simulink model "kcco"  (Simulink 10.0)
settings: Solver=ode45  StartTime=0.0  StopTime=0.05  RelTol=1e-6  EnableMultiTasking=on
settings Model: Creator=mvcmv  LastModifiedBy=mvcmv
settings DataIOCC: LimitDataPoints=on  MaxDataPoints=10000  SignalLoggingSaveFormat=ModelDataLogs  SignalLoggingName=sigsOut
settings OptimizationCC: LifeSpan=auto
settings DebuggingCC: SaveWithParameterizedLinksMsg=none  SignalResolutionControl=TryResolveAllWithWarning  MultiTaskDSMMsg=warning  MultiTaskCondExecSysMsg=none  SFUnexpectedBacktrackingDiag=error  SFNoUnconditionalDefaultTransitionDiag=error  SFExecutionAtInitializationDiag=warning  ArithmeticOperatorsInVariantConditions=error
settings HardwareCC: TargetUnknown=on
settings SFSimCC: SimUseLocalCustomCode=on  CustomCodeUndefinedFunction=FilterOut
settings RTWCC: RTWUseLocalCustomCode=on
settings CodeAppCC: StateflowObjectComments=off
settings GRTTargetCC: TargetLangStandard=C99 (ISO)

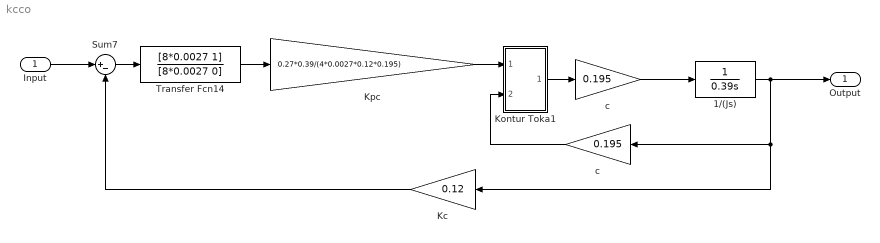
== system kcco ==
  Input : Inport
  1/(Js) : TransferFcn  Denominator=[0.39 0]
  Kc : Gain  Gain=0.12  SaturateOnIntegerOverflow=on  OutDataTypeStr=Inherit: Same as input  ParamDataTypeStr=Inherit: Same as input
  Kontur Toka1 : Subsystem
  Kpc : Gain  Gain=0.27*0.39/(4*0.0027*0.12*0.195)  SaturateOnIntegerOverflow=on  OutDataTypeStr=Inherit: Same as input  ParamDataTypeStr=Inherit: Same as input
  Sum7 : Sum  Inputs=|+-  SaturateOnIntegerOverflow=on
  Transfer Fcn14 : TransferFcn  Numerator=[8*0.0027 1]  Denominator=[8*0.0027 0]
  c : Gain  Gain=0.195  SaturateOnIntegerOverflow=on  OutDataTypeStr=Inherit: Same as input  ParamDataTypeStr=Inherit: Same as input
  с : Gain  Gain=0.195  SaturateOnIntegerOverflow=on  OutDataTypeStr=Inherit: Same as input  ParamDataTypeStr=Inherit: Same as input
  Output : Outport
  wires:
  1/(Js)/1 -> Output/1, с/1, Kc/1
  c/1 -> 1/(Js)/1
  Kontur Toka1/1(Out1) -> c/1
  с/1 -> Kontur Toka1/2(In2)
  Kc/1 -> Sum7/2
  Kpc/1 -> Kontur Toka1/1(In1)
  Transfer Fcn14/1 -> Kpc/1
  Sum7/1 -> Transfer Fcn14/1
  Input/1 -> Sum7/1

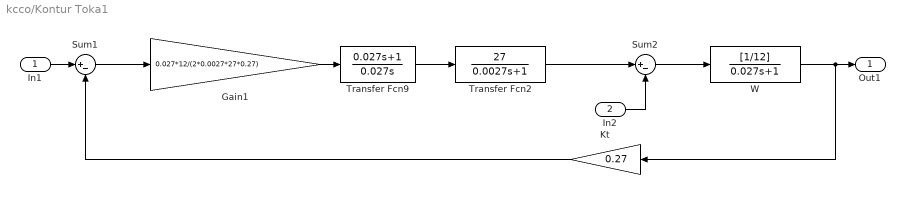
== system kcco/Kontur Toka1 ==
  In1 : Inport
  In2 : Inport  Port=2
  Gain1 : Gain  Gain=0.027*12/(2*0.0027*27*0.27)  SaturateOnIntegerOverflow=on  OutDataTypeStr=Inherit: Same as input  ParamDataTypeStr=Inherit: Same as input
  Kt : Gain  Gain=0.27  SaturateOnIntegerOverflow=on  OutDataTypeStr=Inherit: Same as input  ParamDataTypeStr=Inherit: Same as input
  Sum1 : Sum  Inputs=|+-  SaturateOnIntegerOverflow=on  InputSameDT=on  OutDataTypeStr=Inherit: Same as first input
  Sum2 : Sum  Inputs=|+-  SaturateOnIntegerOverflow=on  InputSameDT=on  OutDataTypeStr=Inherit: Same as first input
  Transfer Fcn2 : TransferFcn  Numerator=[27]  Denominator=[0.0027 1]
  Transfer Fcn9 : TransferFcn  Numerator=[0.027 1]  Denominator=[0.027 0]
  W : TransferFcn  Numerator=[1/12]  Denominator=[0.027 1]
  Out1 : Outport
  wires:
  In2/1 -> Sum2/2
  Sum2/1 -> W/1
  In1/1 -> Sum1/1
  Kt/1 -> Sum1/2
  W/1 -> Kt/1, Out1/1
  Gain1/1 -> Transfer Fcn9/1
  Transfer Fcn9/1 -> Transfer Fcn2/1
  Transfer Fcn2/1 -> Sum2/1
  Sum1/1 -> Gain1/1
